simulink model "teste1"  (R2018a)
settings: Solver=FixedStepAuto  StartTime=0.0  StopTime=22  FixedStep=0.01  RelTol=1e-3
undefined symbols (not defined in the file): C, G
libraries: arduino_io_lib x5
settings Model: Creator=Mauricio  LastModifiedBy=Mauricio

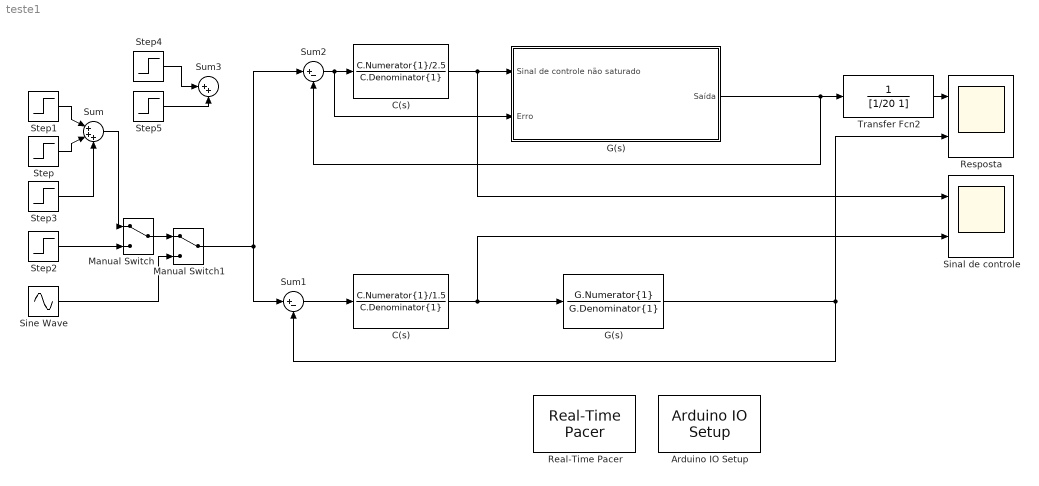
== system teste1 ==
  Arduino IO Setup : arduino_io_lib/Arduino IO Setup  Priority=3  arduinoVar=Temporary arduino variable: Arduino1  workspaceVarName=a  comPort=COM4
  C(s) : TransferFcn  Numerator=C.Numerator{1}/2.5  Denominator=C.Denominator{1}
  "C(s) " : TransferFcn  Numerator=C.Numerator{1}/1.5  Denominator=C.Denominator{1}
  G(s) : TransferFcn  Numerator=G.Numerator{1}  Denominator=G.Denominator{1}
  "G(s) " : Subsystem
  Manual Switch : ManualSwitch
  Manual Switch1 : ManualSwitch
  Real-Time Pacer : arduino_io_lib/Real-Time Pacer  simTimePerRealTime=1
  Resposta : Scope  NumInputPorts=2
  Sinal de controle : Scope  NumInputPorts=2
  Sine Wave : Sin  Amplitude=6  Frequency=2.5  SampleTime=0.05
  Step : Step  Time=10  After=3  SampleTime=0.05
  Step1 : Step  Time=5  After=6  SampleTime=0.05
  Step2 : Step  Time=0  After=0  SampleTime=0.05
  Step3 : Step  Time=15  After=-9  SampleTime=0.05
  Step4 : Step  After=-2  SampleTime=0
  Step5 : Step  Time=10  After=4  SampleTime=0
  Sum : Sum  Inputs=|+++
  Sum1 : Sum  Inputs=|+-
  Sum2 : Sum  Inputs=|+-
  Sum3 : Sum  Inputs=|++
  Transfer Fcn2 : TransferFcn  Denominator=[1/20 1]
  wires:
  Sum2/1 -> "G(s) "/2(Erro), C(s)/1
  C(s)/1 -> Sinal de controle/1, "G(s) "/1(Sinal de controle não saturado)
  Step1/1 -> Sum/1
  Step2/1 -> Manual Switch/2
  Sum1/1 -> "C(s) "/1
  Step/1 -> Sum/2
  Step3/1 -> Sum/3
  Manual Switch/1 -> Manual Switch1/1
  Sine Wave/1 -> Manual Switch1/2
  Manual Switch1/1 -> Sum1/1, Sum2/1
  Step4/1 -> Sum3/1
  Step5/1 -> Sum3/2
  "G(s) "/1(Saída) -> Sum2/2, Transfer Fcn2/1
  G(s)/1 -> Resposta/2, Sum1/2
  "C(s) "/1 -> G(s)/1, Sinal de controle/2
  Sum/1 -> Manual Switch/1
  Transfer Fcn2/1 -> Resposta/1

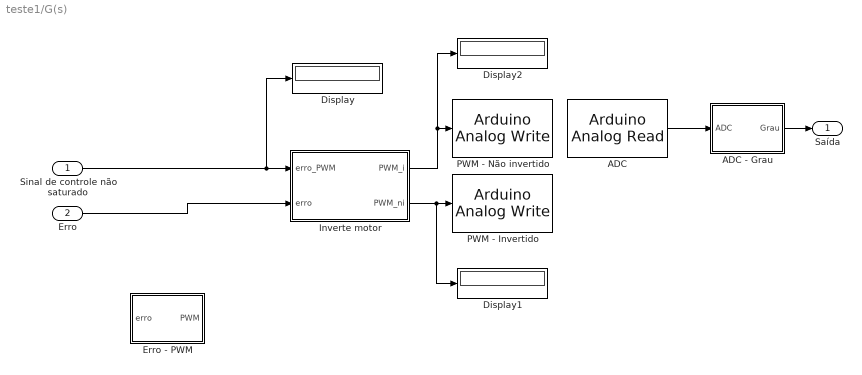
== system teste1/G(s)  ==
  Sinal de controle não saturado : Inport
  Erro : Inport  Port=2
  ADC : arduino_io_lib/Arduino Analog Read  arduinoVar=Temporary arduino variable: Arduino1  arduinoPin=2  T=0.01
  ADC - Grau : MATLAB Function  TreatAsAtomicUnit=on
  Display : Display
  Display1 : Display
  Display2 : Display
  Erro - PWM : MATLAB Function  TreatAsAtomicUnit=on
  Inverte motor : MATLAB Function  TreatAsAtomicUnit=on
  PWM - Invertido : arduino_io_lib/Arduino Analog Write  arduinoVar=Temporary arduino variable: Arduino1  arduinoPin=6  T=0.05
  PWM - Não invertido : arduino_io_lib/Arduino Analog Write  arduinoVar=Temporary arduino variable: Arduino1  arduinoPin=5  T=0.05
  Saída : Outport
  wires:
  ADC/1 -> ADC - Grau/1(ADC)
  Inverte motor/2(PWM_ni) -> Display1/1, PWM - Invertido/1
  Inverte motor/1(PWM_i) -> Display2/1, PWM - Não invertido/1
  ADC - Grau/1(Grau) -> Saída/1
  Erro/1 -> Inverte motor/2(erro)
  Sinal de controle não saturado/1 -> Display/1, Inverte motor/1(erro_PWM)

== matlab function teste1/G(s) /Erro - PWM ==
  data: erro input; PWM output
function PWM = fcn(erro)

if(erro < pi/180 && erro >=0)
    PWM = 0;
elseif(erro > -pi/180 && erro < 0)
    PWM = 0;
else
    PWM = 150.7783671396903180968372495108*erro + 57.368421052631578947368421052632;
end

== matlab function teste1/G(s) /ADC - Grau ==
  data: ADC input; Grau output
function Grau = fcn(ADC)
Grau = -0.17413322126497163269594452616096*ADC + 136.2690584156335364572389157386;

== matlab function teste1/G(s) /Inverte motor ==
  data: PWM_i output; PWM_ni output; erro_PWM input; erro input
function [PWM_i, PWM_ni] = fcn(erro_PWM, erro)
dead_zone = 45;
erro_permissivel = 0.5;

%Confere se a saída está dentro de um erro aceitável, já que não tem
%integrador no controlador
if(abs(erro) <= erro_permissivel)
    erro_PWM = 0;
end

%DESLIGADO
if(erro_PWM == 0)
    PWM_ni = 0;
    PWM_i = 0;
%REVERSO
elseif(erro_PWM>0)
    erro_PWM = erro_PWM + dead_zone; 
    PWM_i = erro_PWM;
    PWM_ni = 0;
%FRENTE
else
    erro_PWM = erro_PWM - dead_zone;
    PWM_ni = abs(erro_PWM);
    PWM_i = 0;
end
